simulink model "PC_CONTROL_STATION"  (R2023b)
settings: Solver=FixedStepAuto  StartTime=0.0  StopTime=inf  RelTol=1e-3  EnableMultiTasking=on
InitFcn:
  | if RUN_MODE~=5
  |     % clear rpi;
  |     rpi = raspberrypi(CAR_IP, 'pi', 'LabControl');
  |     stopModel(rpi,'CAR_CONTROL_SYSTEM')
  |     while isModelRunning(rpi,'CAR_CONTROL_SYSTEM')
  |          stopModel(rpi,'CAR_CONTROL_SYSTEM')
  |     end
  |     runModel(rpi,'CAR_CONTROL_SYSTEM')
  |      while isModelRunning(rpi,'CAR_CONTROL_SYSTEM')==false
  |          runModel(rpi,'CAR_CONTROL_SYSTEM')
  |      end
  |      % clear rpi;
  | end
StopFcn:
  | if RUN_MODE~=5
  |    clear rpi;
  |    rpi = raspberrypi(CAR_IP, 'pi', 'LabControl');
  |    stopModel(rpi,'CAR_CONTROL_SYSTEM')
  |    while isModelRunning(rpi,'CAR_CONTROL_SYSTEM')
  |    end
  |    clear rpi;
  | end
model workspace (MAT data in the model file):
  SL_ROS_VariableLengthArrays_MaxSizes : object (value not decoded)
values from neighbouring files (symbols this model uses):
  data = theClient.GetLastFrameOfData()    [FuncMotive.m]
undefined symbols (not defined in the file or in its folder): CONTROL, CONTROL_INI, data_SL_Info, MD25, MSG, SAMPLING_TIME, Standard_Devices, SYSID_INPUT, TCP_Protocol, UDP_Protocol
libraries: simulink x51, sldrtlib x46, dspsigattribs x7, ros2lib x3, ctrlSharedLib x2, aerolibanimutils x1
(part 2 of 8)

== system PC_CONTROL_STATION/HARDWARE/RT_MONITORING/TCP 106 ==
  Compare To Zero : simulink/Logic and Bit Operations/Compare To Zero  relop=>  OutDataTypeStr=boolean
  Data Store Read : DataStoreRead  DataStoreName=MSG  SampleTime=CONTROL_INI.PARAM.COMM_SAMPLING_TIME  DataStoreElements=MSG.TX_BUFFER(1,1)  IndexOptions=Index vector (dialog)  Indices=1  OutputSizes=1
  MSG_RX : Subsystem  Priority=10
      settings: RTWSystemCode=Nonreusable function  FunctionWithSeparateData=on
  "MSG_TX " : Subsystem  Priority=10
      settings: RTWSystemCode=Nonreusable function  FunctionWithSeparateData=on
  wires:
  Compare To Zero/1 -> "MSG_TX "/Enable
  Data Store Read/1 -> Compare To Zero/1

== system PC_CONTROL_STATION/HARDWARE/RT_MONITORING/TCP 107 ==
  Compare To Zero : simulink/Logic and Bit Operations/Compare To Zero  relop=>  OutDataTypeStr=boolean
  Data Store Read : DataStoreRead  DataStoreName=MSG  SampleTime=CONTROL_INI.PARAM.COMM_SAMPLING_TIME  DataStoreElements=MSG.TX_BUFFER(1,1)  IndexOptions=Index vector (dialog)  Indices=1  OutputSizes=1
  MSG_RX : Subsystem  Priority=10
      settings: RTWSystemCode=Nonreusable function  FunctionWithSeparateData=on
  "MSG_TX " : Subsystem  Priority=10
      settings: RTWSystemCode=Nonreusable function  FunctionWithSeparateData=on
  wires:
  Compare To Zero/1 -> "MSG_TX "/Enable
  Data Store Read/1 -> Compare To Zero/1

== system PC_CONTROL_STATION/HARDWARE/RT_MONITORING/TCP 108 ==
  Compare To Zero : simulink/Logic and Bit Operations/Compare To Zero  relop=>  OutDataTypeStr=boolean
  Data Store Read : DataStoreRead  DataStoreName=MSG  SampleTime=CONTROL_INI.PARAM.COMM_SAMPLING_TIME  DataStoreElements=MSG.TX_BUFFER(1,1)  IndexOptions=Index vector (dialog)  Indices=1  OutputSizes=1
  MSG_RX : Subsystem  Priority=10
      settings: RTWSystemCode=Nonreusable function  FunctionWithSeparateData=on
  "MSG_TX " : Subsystem  Priority=10
      settings: RTWSystemCode=Nonreusable function  FunctionWithSeparateData=on
  wires:
  Compare To Zero/1 -> "MSG_TX "/Enable
  Data Store Read/1 -> Compare To Zero/1

== system PC_CONTROL_STATION/HARDWARE/RT_MONITORING/TCP 109 ==
  Compare To Zero : simulink/Logic and Bit Operations/Compare To Zero  relop=>  OutDataTypeStr=boolean
  Data Store Read : DataStoreRead  DataStoreName=MSG  SampleTime=CONTROL_INI.PARAM.COMM_SAMPLING_TIME  DataStoreElements=MSG.TX_BUFFER(1,1)  IndexOptions=Index vector (dialog)  Indices=1  OutputSizes=1
  MSG_RX : Subsystem  Priority=10
      settings: RTWSystemCode=Nonreusable function  FunctionWithSeparateData=on
  "MSG_TX " : Subsystem  Priority=10
      settings: RTWSystemCode=Nonreusable function  FunctionWithSeparateData=on
  wires:
  Compare To Zero/1 -> "MSG_TX "/Enable
  Data Store Read/1 -> Compare To Zero/1

== system PC_CONTROL_STATION/HARDWARE/RT_MONITORING/TCP 110 ==
  Compare To Zero : simulink/Logic and Bit Operations/Compare To Zero  relop=>  OutDataTypeStr=boolean
  Data Store Read : DataStoreRead  DataStoreName=MSG  SampleTime=CONTROL_INI.PARAM.COMM_SAMPLING_TIME  DataStoreElements=MSG.TX_BUFFER(1,1)  IndexOptions=Index vector (dialog)  Indices=1  OutputSizes=1
  MSG_RX : Subsystem  Priority=10
      settings: RTWSystemCode=Nonreusable function  FunctionWithSeparateData=on
  "MSG_TX " : Subsystem  Priority=10
      settings: RTWSystemCode=Nonreusable function  FunctionWithSeparateData=on
  wires:
  Compare To Zero/1 -> "MSG_TX "/Enable
  Data Store Read/1 -> Compare To Zero/1

== system PC_CONTROL_STATION/HARDWARE/RT_MONITORING/TCP 111 ==
  Compare To Zero : simulink/Logic and Bit Operations/Compare To Zero  relop=>  OutDataTypeStr=boolean
  Data Store Read : DataStoreRead  DataStoreName=MSG  SampleTime=CONTROL_INI.PARAM.COMM_SAMPLING_TIME  DataStoreElements=MSG.TX_BUFFER(1,1)  IndexOptions=Index vector (dialog)  Indices=1  OutputSizes=1
  MSG_RX : Subsystem  Priority=10
      settings: RTWSystemCode=Nonreusable function  FunctionWithSeparateData=on
  "MSG_TX " : Subsystem  Priority=10
      settings: RTWSystemCode=Nonreusable function  FunctionWithSeparateData=on
  wires:
  Compare To Zero/1 -> "MSG_TX "/Enable
  Data Store Read/1 -> Compare To Zero/1

== system PC_CONTROL_STATION/HARDWARE/RT_MONITORING/TCP 112 ==
  Compare To Zero : simulink/Logic and Bit Operations/Compare To Zero  relop=>  OutDataTypeStr=boolean
  Data Store Read : DataStoreRead  DataStoreName=MSG  SampleTime=CONTROL_INI.PARAM.COMM_SAMPLING_TIME  DataStoreElements=MSG.TX_BUFFER(1,1)  IndexOptions=Index vector (dialog)  Indices=1  OutputSizes=1
  MSG_RX : Subsystem  Priority=10
      settings: RTWSystemCode=Nonreusable function  FunctionWithSeparateData=on
  "MSG_TX " : Subsystem  Priority=10
      settings: RTWSystemCode=Nonreusable function  FunctionWithSeparateData=on
  wires:
  Compare To Zero/1 -> "MSG_TX "/Enable
  Data Store Read/1 -> Compare To Zero/1

== system PC_CONTROL_STATION/HARDWARE/RT_MONITORING/TCP 113 ==
  Compare To Zero : simulink/Logic and Bit Operations/Compare To Zero  relop=>  OutDataTypeStr=boolean
  Data Store Read : DataStoreRead  DataStoreName=MSG  SampleTime=CONTROL_INI.PARAM.COMM_SAMPLING_TIME  DataStoreElements=MSG.TX_BUFFER(1,1)  IndexOptions=Index vector (dialog)  Indices=1  OutputSizes=1
  MSG_RX : Subsystem  Priority=10
      settings: RTWSystemCode=Nonreusable function  FunctionWithSeparateData=on
  "MSG_TX " : Subsystem  Priority=10
      settings: RTWSystemCode=Nonreusable function  FunctionWithSeparateData=on
  wires:
  Compare To Zero/1 -> "MSG_TX "/Enable
  Data Store Read/1 -> Compare To Zero/1

== system PC_CONTROL_STATION/HARDWARE/RT_MONITORING/TCP 114 ==
  Compare To Zero : simulink/Logic and Bit Operations/Compare To Zero  relop=>  OutDataTypeStr=boolean
  Data Store Read : DataStoreRead  DataStoreName=MSG  SampleTime=CONTROL_INI.PARAM.COMM_SAMPLING_TIME  DataStoreElements=MSG.TX_BUFFER(1,1)  IndexOptions=Index vector (dialog)  Indices=1  OutputSizes=1
  MSG_RX : Subsystem  Priority=10
      settings: RTWSystemCode=Nonreusable function  FunctionWithSeparateData=on
  "MSG_TX " : Subsystem  Priority=10
      settings: RTWSystemCode=Nonreusable function  FunctionWithSeparateData=on
  wires:
  Compare To Zero/1 -> "MSG_TX "/Enable
  Data Store Read/1 -> Compare To Zero/1

== system PC_CONTROL_STATION/HARDWARE/RT_MONITORING/TCP 115 ==
  Compare To Zero : simulink/Logic and Bit Operations/Compare To Zero  relop=>  OutDataTypeStr=boolean
  Data Store Read : DataStoreRead  DataStoreName=MSG  SampleTime=CONTROL_INI.PARAM.COMM_SAMPLING_TIME  DataStoreElements=MSG.TX_BUFFER(1,1)  IndexOptions=Index vector (dialog)  Indices=1  OutputSizes=1
  MSG_RX : Subsystem  Priority=10
      settings: RTWSystemCode=Nonreusable function  FunctionWithSeparateData=on
  "MSG_TX " : Subsystem  Priority=10
      settings: RTWSystemCode=Nonreusable function  FunctionWithSeparateData=on
  wires:
  Compare To Zero/1 -> "MSG_TX "/Enable
  Data Store Read/1 -> Compare To Zero/1

== system PC_CONTROL_STATION/HARDWARE/RT_MONITORING/TCP 116 ==
  Compare To Zero : simulink/Logic and Bit Operations/Compare To Zero  relop=>  OutDataTypeStr=boolean
  Data Store Read : DataStoreRead  DataStoreName=MSG  SampleTime=CONTROL_INI.PARAM.COMM_SAMPLING_TIME  DataStoreElements=MSG.TX_BUFFER(1,1)  IndexOptions=Index vector (dialog)  Indices=1  OutputSizes=1
  MSG_RX : Subsystem  Priority=10
      settings: RTWSystemCode=Nonreusable function  FunctionWithSeparateData=on
  "MSG_TX " : Subsystem  Priority=10
      settings: RTWSystemCode=Nonreusable function  FunctionWithSeparateData=on
  wires:
  Compare To Zero/1 -> "MSG_TX "/Enable
  Data Store Read/1 -> Compare To Zero/1

== system PC_CONTROL_STATION/HARDWARE/RT_MONITORING/TCP 117 ==
  Compare To Zero : simulink/Logic and Bit Operations/Compare To Zero  relop=>  OutDataTypeStr=boolean
  Data Store Read : DataStoreRead  DataStoreName=MSG  SampleTime=CONTROL_INI.PARAM.COMM_SAMPLING_TIME  DataStoreElements=MSG.TX_BUFFER(1,1)  IndexOptions=Index vector (dialog)  Indices=1  OutputSizes=1
  MSG_RX : Subsystem  Priority=10
      settings: RTWSystemCode=Nonreusable function  FunctionWithSeparateData=on
  "MSG_TX " : Subsystem  Priority=10
      settings: RTWSystemCode=Nonreusable function  FunctionWithSeparateData=on
  wires:
  Compare To Zero/1 -> "MSG_TX "/Enable
  Data Store Read/1 -> Compare To Zero/1

== system PC_CONTROL_STATION/HARDWARE/RT_MONITORING/TCP 118 ==
  Compare To Zero : simulink/Logic and Bit Operations/Compare To Zero  relop=>  OutDataTypeStr=boolean
  Data Store Read : DataStoreRead  DataStoreName=MSG  SampleTime=CONTROL_INI.PARAM.COMM_SAMPLING_TIME  DataStoreElements=MSG.TX_BUFFER(1,1)  IndexOptions=Index vector (dialog)  Indices=1  OutputSizes=1
  MSG_RX : Subsystem  Priority=10
      settings: RTWSystemCode=Nonreusable function  FunctionWithSeparateData=on
  "MSG_TX " : Subsystem  Priority=10
      settings: RTWSystemCode=Nonreusable function  FunctionWithSeparateData=on
  wires:
  Compare To Zero/1 -> "MSG_TX "/Enable
  Data Store Read/1 -> Compare To Zero/1

== system PC_CONTROL_STATION/HARDWARE/RT_MONITORING/TCP 119 ==
  Compare To Zero : simulink/Logic and Bit Operations/Compare To Zero  relop=>  OutDataTypeStr=boolean
  Data Store Read : DataStoreRead  DataStoreName=MSG  SampleTime=CONTROL_INI.PARAM.COMM_SAMPLING_TIME  DataStoreElements=MSG.TX_BUFFER(1,1)  IndexOptions=Index vector (dialog)  Indices=1  OutputSizes=1
  MSG_RX : Subsystem  Priority=10
      settings: RTWSystemCode=Nonreusable function  FunctionWithSeparateData=on
  "MSG_TX " : Subsystem  Priority=10
      settings: RTWSystemCode=Nonreusable function  FunctionWithSeparateData=on
  wires:
  Compare To Zero/1 -> "MSG_TX "/Enable
  Data Store Read/1 -> Compare To Zero/1

== system PC_CONTROL_STATION/HARDWARE/RT_MONITORING/TCP 120 ==
  Compare To Zero : simulink/Logic and Bit Operations/Compare To Zero  relop=>  OutDataTypeStr=boolean
  Data Store Read : DataStoreRead  DataStoreName=MSG  SampleTime=CONTROL_INI.PARAM.COMM_SAMPLING_TIME  DataStoreElements=MSG.TX_BUFFER(1,1)  IndexOptions=Index vector (dialog)  Indices=1  OutputSizes=1
  MSG_RX : Subsystem  Priority=10
      settings: RTWSystemCode=Nonreusable function  FunctionWithSeparateData=on
  "MSG_TX " : Subsystem  Priority=10
      settings: RTWSystemCode=Nonreusable function  FunctionWithSeparateData=on
  wires:
  Compare To Zero/1 -> "MSG_TX "/Enable
  Data Store Read/1 -> Compare To Zero/1

== system PC_CONTROL_STATION/HARDWARE/RT_MONITORING/TCP 121 ==
  Compare To Zero : simulink/Logic and Bit Operations/Compare To Zero  relop=>  OutDataTypeStr=boolean
  Data Store Read : DataStoreRead  DataStoreName=MSG  SampleTime=CONTROL_INI.PARAM.COMM_SAMPLING_TIME  DataStoreElements=MSG.TX_BUFFER(1,1)  IndexOptions=Index vector (dialog)  Indices=1  OutputSizes=1
  MSG_RX : Subsystem  Priority=10
      settings: RTWSystemCode=Nonreusable function  FunctionWithSeparateData=on
  "MSG_TX " : Subsystem  Priority=10
      settings: RTWSystemCode=Nonreusable function  FunctionWithSeparateData=on
  wires:
  Compare To Zero/1 -> "MSG_TX "/Enable
  Data Store Read/1 -> Compare To Zero/1

== system PC_CONTROL_STATION/HARDWARE/RT_MONITORING/TCP RSP ==
  Compare To Zero : simulink/Logic and Bit Operations/Compare To Zero  relop=>  OutDataTypeStr=boolean
  Data Store Read : DataStoreRead  DataStoreName=MSG  SampleTime=CONTROL_INI.PARAM.COMM_SAMPLING_TIME  DataStoreElements=MSG.TX_BUFFER(1,1)  IndexOptions=Index vector (dialog)  Indices=1  OutputSizes=1
  MSG_RX : Subsystem  Priority=10
      settings: RTWSystemCode=Nonreusable function  FunctionWithSeparateData=on
  "MSG_TX " : Subsystem  Priority=10
      settings: RTWSystemCode=Nonreusable function  FunctionWithSeparateData=on
  wires:
  Compare To Zero/1 -> "MSG_TX "/Enable
  Data Store Read/1 -> Compare To Zero/1

== system PC_CONTROL_STATION/HARDWARE/RT_MONITORING/UDP ==
  Compare To Zero : simulink/Logic and Bit Operations/Compare To Zero  relop=>  OutDataTypeStr=boolean
  Data Store Read : DataStoreRead  DataStoreName=MSG  SampleTime=CONTROL_INI.PARAM.COMM_SAMPLING_TIME  DataStoreElements=MSG.TX_BUFFER(1,1)  IndexOptions=Index vector (dialog)  Indices=1  OutputSizes=1
  MSG_RX : Subsystem  Priority=10
      settings: RTWSystemCode=Nonreusable function  FunctionWithSeparateData=on
  "MSG_TX " : Subsystem  Priority=10
      settings: RTWSystemCode=Nonreusable function  FunctionWithSeparateData=on
  wires:
  Compare To Zero/1 -> "MSG_TX "/Enable
  Data Store Read/1 -> Compare To Zero/1

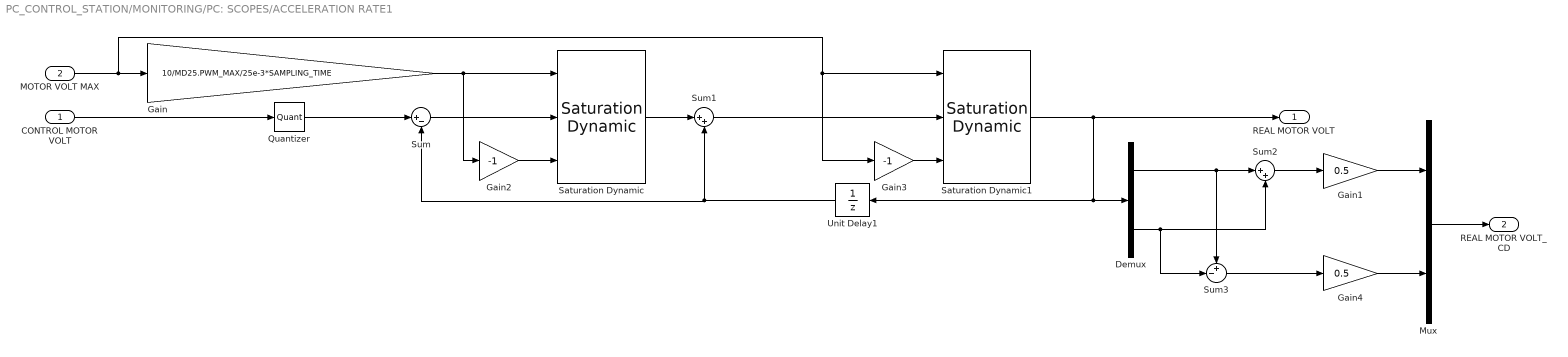
== system PC_CONTROL_STATION/MONITORING/PC: SCOPES/ACCELERATION RATE1 ==
  CONTROL MOTOR VOLT : Inport
  MOTOR VOLT MAX : Inport  Port=2
  Demux : Demux  Outputs=2
  Gain : Gain  Gain=10/MD25.PWM_MAX/25e-3*SAMPLING_TIME
  Gain1 : Gain  Gain=0.5
  Gain2 : Gain  Gain=-1
  Gain3 : Gain  Gain=-1
  Gain4 : Gain  Gain=0.5
  Mux : Mux  Inputs=2
  Quantizer : Quantizer  QuantizationInterval=CONTROL_INI.PARAM.MOTOR_VOLT_MAX(1)/127
  Saturation Dynamic : simulink/Discontinuities/Saturation Dynamic  OutMin=[]  OutMax=[]  OutDataTypeStr=Inherit: Same as second input  OutDataType=fixdt(1, 16)  OutScaling=2^-10  DoSatur=off
  Saturation Dynamic1 : simulink/Discontinuities/Saturation Dynamic  OutMin=[]  OutMax=[]  OutDataTypeStr=Inherit: Same as second input  OutDataType=fixdt(1, 16)  OutScaling=2^-10  DoSatur=off
  Sum : Sum  Inputs=|+-
  Sum1 : Sum  Inputs=|++
  Sum2 : Sum  Inputs=|++
  Sum3 : Sum  Inputs=+-|
  Unit Delay1 : UnitDelay  SampleTime=-1  HasFrameUpgradeWarning=on
  REAL MOTOR VOLT : Outport
  REAL MOTOR VOLT_CD : Outport  Port=2
  wires:
  CONTROL MOTOR VOLT/1 -> Quantizer/1
  Gain3/1 -> Saturation Dynamic1/3
  Gain2/1 -> Saturation Dynamic/3
  Sum/1 -> Saturation Dynamic/2
  MOTOR VOLT MAX/1 -> Gain/1, Gain3/1, Saturation Dynamic1/1
  Sum1/1 -> Saturation Dynamic1/2
  Gain/1 -> Gain2/1, Saturation Dynamic/1
  Saturation Dynamic/1 -> Sum1/1
  Saturation Dynamic1/1 -> Unit Delay1/1, Demux/1, REAL MOTOR VOLT/1
  Demux/1 -> Sum3/1, Sum2/1
  Demux/2 -> Sum3/2, Sum2/2
  Sum2/1 -> Gain1/1
  Sum3/1 -> Gain4/1
  Gain1/1 -> Mux/1
  Gain4/1 -> Mux/2
  Mux/1 -> REAL MOTOR VOLT_CD/1
  Unit Delay1/1 -> Sum/2, Sum1/2
  Quantizer/1 -> Sum/1

== system PC_CONTROL_STATION/MONITORING/SYSTEM IDENTIFICATION/STATE VARIABLE FILTER 1 ==
  IN : Inport
  Add : Sum  Inputs=3
  Constant : Constant  Value=SVF_B1d  SampleTime=SAMPLING_TIME
  Constant1 : Constant  Value=SVF_B2d  SampleTime=SAMPLING_TIME
  Constant2 : Constant  Value=SVF_Ad  SampleTime=SAMPLING_TIME
  Divide : Product  Multiplication=Matrix(*)
  Divide1 : Product  Multiplication=Matrix(*)
  Divide2 : Product  Multiplication=Matrix(*)
  Unit Delay : UnitDelay  InitialCondition=zeros(4,1)  SampleTime=-1  HasFrameUpgradeWarning=on
  Unit Delay1 : UnitDelay  SampleTime=-1  HasFrameUpgradeWarning=on
  STATE : Outport  VectorParamsAs1DForOutWhenUnconnected=off
  wires:
  Constant/1 -> Divide1/1
  Unit Delay1/1 -> Divide1/2
  Divide1/1 -> Add/1
  Add/1 -> STATE/1, Unit Delay/1
  Divide/1 -> Add/2
  Constant1/1 -> Divide/1
  Divide2/1 -> Add/3
  Constant2/1 -> Divide2/1
  Unit Delay/1 -> Divide2/2
  IN/1 -> Divide/2, Unit Delay1/1

== system PC_CONTROL_STATION/MONITORING/SYSTEM IDENTIFICATION/STATE VARIABLE FILTER 2 ==
  IN : Inport
  Add : Sum  Inputs=3
  Constant : Constant  Value=SVF_B1d  SampleTime=SAMPLING_TIME
  Constant1 : Constant  Value=SVF_B2d  SampleTime=SAMPLING_TIME
  Constant2 : Constant  Value=SVF_Ad  SampleTime=SAMPLING_TIME
  Divide : Product  Multiplication=Matrix(*)
  Divide1 : Product  Multiplication=Matrix(*)
  Divide2 : Product  Multiplication=Matrix(*)
  Unit Delay : UnitDelay  InitialCondition=zeros(4,1)  SampleTime=-1  HasFrameUpgradeWarning=on
  Unit Delay1 : UnitDelay  SampleTime=-1  HasFrameUpgradeWarning=on
  STATE : Outport  VectorParamsAs1DForOutWhenUnconnected=off
  wires:
  IN/1 -> Unit Delay1/1, Divide/2
  Unit Delay/1 -> Divide2/2
  Constant2/1 -> Divide2/1
  Divide2/1 -> Add/3
  Constant1/1 -> Divide/1
  Divide/1 -> Add/2
  Add/1 -> Unit Delay/1, STATE/1
  Divide1/1 -> Add/1
  Unit Delay1/1 -> Divide1/2
  Constant/1 -> Divide1/1

== system PC_CONTROL_STATION/MONITORING/SYSTEM IDENTIFICATION/STATE VARIABLE FILTER 3 ==
  IN : Inport
  Add : Sum  Inputs=3
  Constant : Constant  Value=SVF_B1d  SampleTime=SAMPLING_TIME
  Constant1 : Constant  Value=SVF_B2d  SampleTime=SAMPLING_TIME
  Constant2 : Constant  Value=SVF_Ad  SampleTime=SAMPLING_TIME
  Divide : Product  Multiplication=Matrix(*)
  Divide1 : Product  Multiplication=Matrix(*)
  Divide2 : Product  Multiplication=Matrix(*)
  Unit Delay : UnitDelay  InitialCondition=zeros(4,1)  SampleTime=-1  HasFrameUpgradeWarning=on
  Unit Delay1 : UnitDelay  SampleTime=-1  HasFrameUpgradeWarning=on
  STATE : Outport  VectorParamsAs1DForOutWhenUnconnected=off
  wires:
  Constant/1 -> Divide1/1
  Unit Delay1/1 -> Divide1/2
  Divide1/1 -> Add/1
  Add/1 -> STATE/1, Unit Delay/1
  Divide/1 -> Add/2
  Constant1/1 -> Divide/1
  Divide2/1 -> Add/3
  Constant2/1 -> Divide2/1
  Unit Delay/1 -> Divide2/2
  IN/1 -> Divide/2, Unit Delay1/1

== system PC_CONTROL_STATION/MONITORING/SYSTEM IDENTIFICATION/STATE VARIABLE FILTER 4 ==
  IN : Inport
  Add : Sum  Inputs=3
  Constant : Constant  Value=SVF_B1d  SampleTime=SAMPLING_TIME
  Constant1 : Constant  Value=SVF_B2d  SampleTime=SAMPLING_TIME
  Constant2 : Constant  Value=SVF_Ad  SampleTime=SAMPLING_TIME
  Divide : Product  Multiplication=Matrix(*)
  Divide1 : Product  Multiplication=Matrix(*)
  Divide2 : Product  Multiplication=Matrix(*)
  Unit Delay : UnitDelay  InitialCondition=zeros(4,1)  SampleTime=-1  HasFrameUpgradeWarning=on
  Unit Delay1 : UnitDelay  SampleTime=-1  HasFrameUpgradeWarning=on
  STATE : Outport  VectorParamsAs1DForOutWhenUnconnected=off
  wires:
  IN/1 -> Unit Delay1/1, Divide/2
  Unit Delay/1 -> Divide2/2
  Constant2/1 -> Divide2/1
  Divide2/1 -> Add/3
  Constant1/1 -> Divide/1
  Divide/1 -> Add/2
  Add/1 -> Unit Delay/1, STATE/1
  Divide1/1 -> Add/1
  Unit Delay1/1 -> Divide1/2
  Constant/1 -> Divide1/1

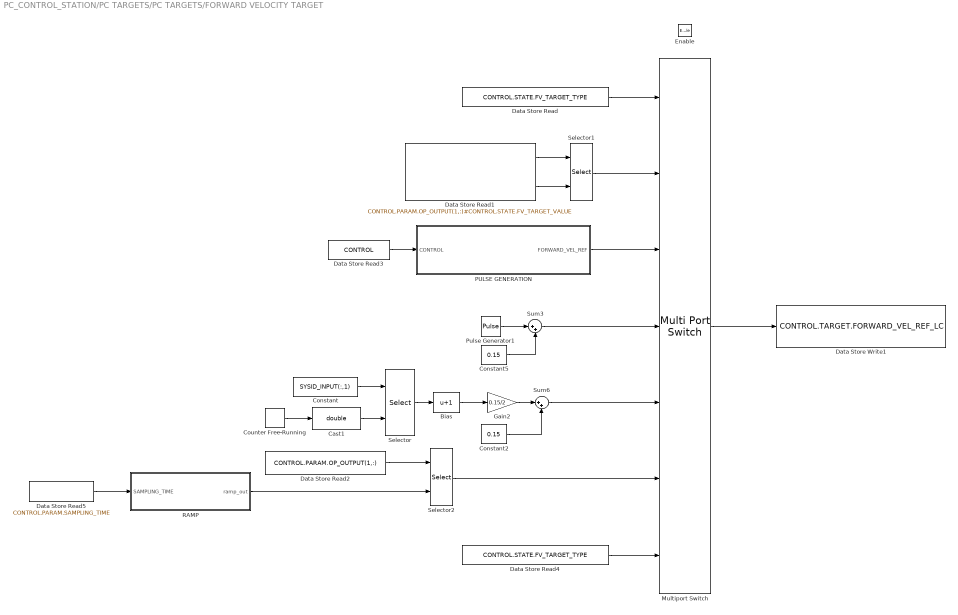
== system PC_CONTROL_STATION/PC TARGETS/PC TARGETS/FORWARD VELOCITY TARGET ==
  Enable : EnablePort
  " PULSE GENERATION" : MATLAB Function  Priority=60  TreatAsAtomicUnit=on
  Bias : Bias  Bias=1  SaturateOnIntegerOverflow=off
  Cast1 : DataTypeConversion  OutDataTypeStr=double  SaturateOnIntegerOverflow=off  RndMeth=Floor
  Constant : Constant  Value=SYSID_INPUT(:,1)  SampleTime=SAMPLING_TIME
  Constant2 : Constant  Value=0.15  OutDataTypeStr=double  SampleTime=SAMPLING_TIME
  Constant5 : Constant  Value=0.15  OutDataTypeStr=double  SampleTime=SAMPLING_TIME
  Counter Free-Running : simulink/Sources/Counter Free-Running  NumBits=9  tsamp=SAMPLING_TIME
  Data Store Read : DataStoreRead  DataStoreName=CONTROL  SampleTime=SAMPLING_TIME  DataStoreElements=CONTROL.STATE.FV_TARGET_TYPE  IndexOptions=Index vector (dialog)  Indices=1  OutputSizes=1
  Data Store Read1 : DataStoreRead  DataStoreName=CONTROL  SampleTime=SAMPLING_TIME  DataStoreElements=CONTROL.PARAM.OP_OUTPUT(1,:)#CONTROL.STATE.FV_TARGET_VALUE  IndexOptions=Index vector (dialog)  Indices=1  OutputSizes=1
  Data Store Read2 : DataStoreRead  DataStoreName=CONTROL  SampleTime=SAMPLING_TIME  DataStoreElements=CONTROL.PARAM.OP_OUTPUT(1,:)  IndexOptions=Index vector (dialog)  Indices=1  OutputSizes=1
  Data Store Read3 : DataStoreRead  DataStoreName=CONTROL  SampleTime=SAMPLING_TIME  IndexOptions=Index vector (dialog)  Indices=1  OutputSizes=1
  Data Store Read4 : DataStoreRead  DataStoreName=CONTROL  SampleTime=SAMPLING_TIME  DataStoreElements=CONTROL.STATE.FV_TARGET_TYPE  IndexOptions=Index vector (dialog)  Indices=1  OutputSizes=1
  Data Store Read5 : DataStoreRead  DataStoreName=CONTROL  SampleTime=SAMPLING_TIME  DataStoreElements=CONTROL.PARAM.SAMPLING_TIME  IndexOptions=Index vector (dialog)  Indices=1  OutputSizes=1
  Data Store Write1 : DataStoreWrite  DataStoreName=CONTROL  SampleTime=SAMPLING_TIME  DataStoreElements=CONTROL.TARGET.FORWARD_VEL_REF_LC  IndexOptions=Index vector (dialog)  Indices=1  OutputSizes=1
  Gain2 : Gain  Gain=0.15/2
  Multiport Switch : MultiPortSwitch  DataPortOrder=Zero-based contiguous  Inputs=6  zeroidx=on  SaturateOnIntegerOverflow=off  InputSameDT=off
  Pulse Generator1 : DiscretePulseGenerator  Amplitude=0.15  Period=500  PulseWidth=250  SampleTime=SAMPLING_TIME
  RAMP : MATLAB Function  TreatAsAtomicUnit=on
  Selector : Selector  IndexMode=Zero-based  InputPortWidth=512  IndexOptions=Index vector (port)  Indices=[1 3]  OutputSizes=1
  Selector1 : Selector  InputPortWidth=4  IndexOptions=Index vector (port)  Indices=[1 3]  OutputSizes=1
  Selector2 : Selector  InputPortWidth=4  IndexOptions=Index vector (port)  Indices=[1 3]  OutputSizes=1
  Sum3 : Sum  Inputs=|++
  Sum6 : Sum  Inputs=|++
  wires:
  Constant5/1 -> Sum3/2
  Pulse Generator1/1 -> Sum3/1
  Counter Free-Running/1 -> Cast1/1
  Sum6/1 -> Multiport Switch/5
  Sum3/1 -> Multiport Switch/4
  Gain2/1 -> Sum6/1
  Selector1/1 -> Multiport Switch/2
  Constant/1 -> Selector/1
  Data Store Read/1 -> Multiport Switch/1
  Cast1/1 -> Selector/2
  Constant2/1 -> Sum6/2
  Multiport Switch/1 -> Data Store Write1/1
  Data Store Read3/1 -> " PULSE GENERATION"/1(CONTROL)
  " PULSE GENERATION"/1(FORWARD_VEL_REF) -> Multiport Switch/3
  Data Store Read1/1 -> Selector1/1
  Data Store Read1/2 -> Selector1/2
  Selector2/1 -> Multiport Switch/6
  Data Store Read2/1 -> Selector2/1
  Data Store Read4/1 -> Multiport Switch/7
  RAMP/1(ramp_out) -> Selector2/2
  Data Store Read5/1 -> RAMP/1(SAMPLING_TIME)
  Selector/1 -> Bias/1
  Bias/1 -> Gain2/1

== system PC_CONTROL_STATION/PC TARGETS/PC TARGETS/NAVIGATION TARGETS ==
  Enable : EnablePort
  Data Store Read7 : DataStoreRead  DataStoreName=CONTROL  SampleTime=SAMPLING_TIME  IndexOptions=Index vector (dialog)  Indices=1  OutputSizes=1
  Data Store Write : DataStoreWrite  DataStoreName=CONTROL  SampleTime=SAMPLING_TIME  IndexOptions=Index vector (dialog)  Indices=1  OutputSizes=1
  TRAJECTORY PLANNER (POLYNOMIAL IN Vx & Vy) : MATLAB Function  Priority=10  TreatAsAtomicUnit=on
  wires:
  Data Store Read7/1 -> TRAJECTORY PLANNER (POLYNOMIAL IN Vx & Vy)/1(CONTROL_IN)
  TRAJECTORY PLANNER (POLYNOMIAL IN Vx & Vy)/1(CONTROL) -> Data Store Write/1

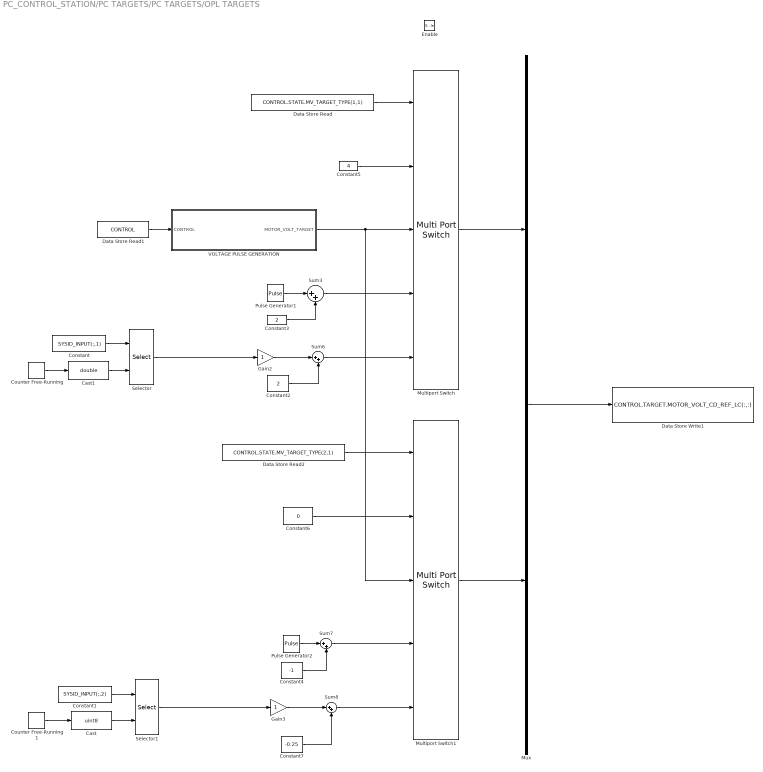
== system PC_CONTROL_STATION/PC TARGETS/PC TARGETS/OPL TARGETS ==
  Enable : EnablePort
  Cast : DataTypeConversion  OutDataTypeStr=uint8  SaturateOnIntegerOverflow=off  RndMeth=Floor
  Cast1 : DataTypeConversion  OutDataTypeStr=double  SaturateOnIntegerOverflow=off  RndMeth=Floor
  Constant : Constant  Value=SYSID_INPUT(:,1)  SampleTime=SAMPLING_TIME
  Constant1 : Constant  Value=SYSID_INPUT(:,2)  SampleTime=SAMPLING_TIME
  Constant2 : Constant  Value=2  OutDataTypeStr=single  SampleTime=SAMPLING_TIME
  Constant3 : Constant  Value=2  OutDataTypeStr=double  SampleTime=SAMPLING_TIME
  Constant4 : Constant  Value=-1  OutDataTypeStr=single  SampleTime=SAMPLING_TIME
  Constant5 : Constant  Value=4  OutDataTypeStr=double  SampleTime=SAMPLING_TIME
  Constant6 : Constant  Value=0  OutDataTypeStr=double  SampleTime=SAMPLING_TIME
  Constant7 : Constant  Value=-0.25  OutDataTypeStr=single  SampleTime=SAMPLING_TIME
  Counter Free-Running : simulink/Sources/Counter Free-Running  NumBits=9  tsamp=SAMPLING_TIME
  Counter Free-Running1 : simulink/Sources/Counter Free-Running  NumBits=9  tsamp=SAMPLING_TIME
  Data Store Read : DataStoreRead  DataStoreName=CONTROL  SampleTime=SAMPLING_TIME  DataStoreElements=CONTROL.STATE.MV_TARGET_TYPE(1,1)  IndexOptions=Index vector (dialog)  Indices=1  OutputSizes=1
  Data Store Read1 : DataStoreRead  DataStoreName=CONTROL  SampleTime=SAMPLING_TIME  IndexOptions=Index vector (dialog)  Indices=1  OutputSizes=1
  Data Store Read2 : DataStoreRead  DataStoreName=CONTROL  SampleTime=SAMPLING_TIME  DataStoreElements=CONTROL.STATE.MV_TARGET_TYPE(2,1)  IndexOptions=Index vector (dialog)  Indices=1  OutputSizes=1
  Data Store Write1 : DataStoreWrite  DataStoreName=CONTROL  SampleTime=SAMPLING_TIME  DataStoreElements=CONTROL.TARGET.MOTOR_VOLT_CD_REF_LC(:,:)  IndexOptions=Index vector (dialog)  Indices=1  OutputSizes=1
  Gain2 : Gain
  Gain3 : Gain
  Multiport Switch : MultiPortSwitch  DataPortOrder=Zero-based contiguous  Inputs=4  zeroidx=on  SaturateOnIntegerOverflow=off  InputSameDT=off
  Multiport Switch1 : MultiPortSwitch  DataPortOrder=Zero-based contiguous  Inputs=4  zeroidx=on  SaturateOnIntegerOverflow=off  InputSameDT=off
  Mux : Mux  Inputs=2
  Pulse Generator1 : DiscretePulseGenerator  Amplitude=2  Period=200  PulseWidth=100  SampleTime=SAMPLING_TIME
  Pulse Generator2 : DiscretePulseGenerator  Amplitude=2  Period=200  PulseWidth=100  SampleTime=SAMPLING_TIME
  Selector : Selector  IndexMode=Zero-based  InputPortWidth=512  IndexOptions=Index vector (port)  Indices=[1 3]  OutputSizes=1
  Selector1 : Selector  IndexMode=Zero-based  InputPortWidth=512  IndexOptions=Index vector (port)  Indices=[1 3]  OutputSizes=1
  Sum{3,6..8} (4 alike) : Sum  Inputs=|++
  VOLTAGE PULSE GENERATION : MATLAB Function  Priority=60  TreatAsAtomicUnit=on
  wires:
  VOLTAGE PULSE GENERATION/1(MOTOR_VOLT_TARGET) -> Multiport Switch/3, Multiport Switch1/3
  Constant6/1 -> Multiport Switch1/2
  Constant7/1 -> Sum8/2
  Sum6/1 -> Multiport Switch/5
  Mux/1 -> Data Store Write1/1
  Sum3/1 -> Multiport Switch/4
  Gain2/1 -> Sum6/1
  Counter Free-Running/1 -> Cast1/1
  Cast1/1 -> Selector/2
  Sum8/1 -> Multiport Switch1/5
  Sum7/1 -> Multiport Switch1/4
  Selector1/1 -> Gain3/1
  Multiport Switch1/1 -> Mux/2
  Constant1/1 -> Selector1/1
  Constant/1 -> Selector/1
  Constant4/1 -> Sum7/2
  Gain3/1 -> Sum8/1
  Multiport Switch/1 -> Mux/1
  Data Store Read2/1 -> Multiport Switch1/1
  Cast/1 -> Selector1/2
  Constant2/1 -> Sum6/2
  Selector/1 -> Gain2/1
  Pulse Generator2/1 -> Sum7/1
  Counter Free-Running1/1 -> Cast/1
  Data Store Read/1 -> Multiport Switch/1
  Data Store Read1/1 -> VOLTAGE PULSE GENERATION/1(CONTROL)
  Constant5/1 -> Multiport Switch/2
  Pulse Generator1/1 -> Sum3/1
  Constant3/1 -> Sum3/2

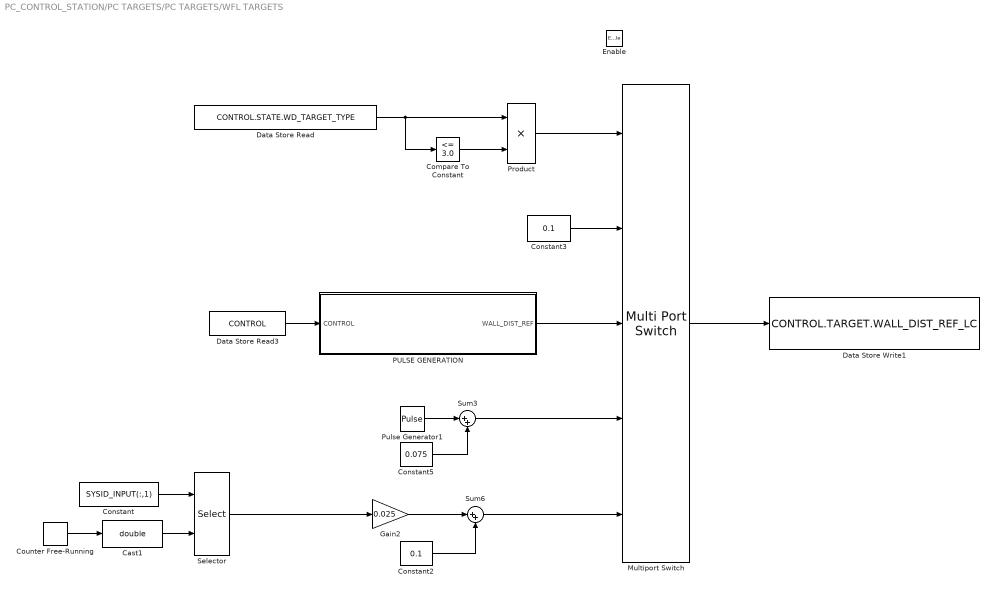
== system PC_CONTROL_STATION/PC TARGETS/PC TARGETS/WFL TARGETS ==
  Enable : EnablePort
  " PULSE GENERATION" : MATLAB Function  Priority=60  TreatAsAtomicUnit=on
  Cast1 : DataTypeConversion  OutDataTypeStr=double  SaturateOnIntegerOverflow=off  RndMeth=Floor
  Compare To Constant : simulink/Logic and Bit Operations/Compare To Constant  relop=<=  const=3.0  OutDataTypeStr=uint8
  Constant : Constant  Value=SYSID_INPUT(:,1)  SampleTime=SAMPLING_TIME
  Constant2 : Constant  Value=0.1  OutDataTypeStr=single  SampleTime=SAMPLING_TIME
  Constant3 : Constant  Value=0.1  OutDataTypeStr=double  SampleTime=SAMPLING_TIME
  Constant5 : Constant  Value=0.075  OutDataTypeStr=single  SampleTime=SAMPLING_TIME
  Counter Free-Running : simulink/Sources/Counter Free-Running  NumBits=9  tsamp=SAMPLING_TIME
  Data Store Read : DataStoreRead  DataStoreName=CONTROL  SampleTime=SAMPLING_TIME  DataStoreElements=CONTROL.STATE.WD_TARGET_TYPE  IndexOptions=Index vector (dialog)  Indices=1  OutputSizes=1
  Data Store Read3 : DataStoreRead  DataStoreName=CONTROL  SampleTime=SAMPLING_TIME  IndexOptions=Index vector (dialog)  Indices=1  OutputSizes=1
  Data Store Write1 : DataStoreWrite  DataStoreName=CONTROL  SampleTime=SAMPLING_TIME  DataStoreElements=CONTROL.TARGET.WALL_DIST_REF_LC  IndexOptions=Index vector (dialog)  Indices=1  OutputSizes=1
  Gain2 : Gain  Gain=0.025
  Multiport Switch : MultiPortSwitch  DataPortOrder=Zero-based contiguous  Inputs=4  zeroidx=on  SaturateOnIntegerOverflow=off  InputSameDT=off
  Product : Product
  Pulse Generator1 : DiscretePulseGenerator  Amplitude=0.025  Period=1000  PulseWidth=500  SampleTime=SAMPLING_TIME
  Selector : Selector  IndexMode=Zero-based  InputPortWidth=512  IndexOptions=Index vector (port)  Indices=[1 3]  OutputSizes=1
  Sum3 : Sum  Inputs=|++
  Sum6 : Sum  Inputs=|++
  wires:
  Pulse Generator1/1 -> Sum3/1
  Data Store Read3/1 -> " PULSE GENERATION"/1(CONTROL)
  Sum6/1 -> Multiport Switch/5
  Sum3/1 -> Multiport Switch/4
  Constant/1 -> Selector/1
  " PULSE GENERATION"/1(WALL_DIST_REF) -> Multiport Switch/3
  Constant2/1 -> Sum6/2
  Gain2/1 -> Sum6/1
  Constant5/1 -> Sum3/2
  Multiport Switch/1 -> Data Store Write1/1
  Cast1/1 -> Selector/2
  Constant3/1 -> Multiport Switch/2
  Selector/1 -> Gain2/1
  Counter Free-Running/1 -> Cast1/1
  Product/1 -> Multiport Switch/1
  Data Store Read/1 -> Compare To Constant/1, Product/1
  Compare To Constant/1 -> Product/2

== system PC_CONTROL_STATION/PC TARGETS/PC TARGETS/YAW ANGLE TARGET ==
  Enable : EnablePort
  " PULSE GENERATION" : MATLAB Function  Priority=60  TreatAsAtomicUnit=on
  Cast1 : DataTypeConversion  OutDataTypeStr=double  SaturateOnIntegerOverflow=off  RndMeth=Floor
  Constant : Constant  Value=SYSID_INPUT(:,1)  SampleTime=SAMPLING_TIME
  Constant3 : Constant  Value=0  OutDataTypeStr=double  SampleTime=SAMPLING_TIME
  Constant5 : Constant  Value=-60*pi/180  OutDataTypeStr=single  SampleTime=SAMPLING_TIME
  Constant8 : Constant  Value=-60*pi/180  OutDataTypeStr=single  SampleTime=SAMPLING_TIME
  Counter Free-Running : simulink/Sources/Counter Free-Running  NumBits=9  tsamp=SAMPLING_TIME
  Data Store Read : DataStoreRead  DataStoreName=CONTROL  SampleTime=SAMPLING_TIME  DataStoreElements=CONTROL.STATE.YA_TARGET_TYPE  IndexOptions=Index vector (dialog)  Indices=1  OutputSizes=1
  Data Store Read1 : DataStoreRead  DataStoreName=CONTROL  SampleTime=SAMPLING_TIME  IndexOptions=Index vector (dialog)  Indices=1  OutputSizes=1
  Data Store Write1 : DataStoreWrite  DataStoreName=CONTROL  SampleTime=SAMPLING_TIME  DataStoreElements=CONTROL.TARGET.YAW_ANG_REF_LC  IndexOptions=Index vector (dialog)  Indices=1  OutputSizes=1
  Gain2 : Gain  Gain=120*pi/180
  Multiport Switch : MultiPortSwitch  DataPortOrder=Zero-based contiguous  Inputs=4  zeroidx=on  SaturateOnIntegerOverflow=off  InputSameDT=off
  Pulse Generator1 : DiscretePulseGenerator  Amplitude=120*pi/180  Period=500  PulseWidth=250  PhaseDelay=125  SampleTime=SAMPLING_TIME
  Selector : Selector  IndexMode=Zero-based  InputPortWidth=512  IndexOptions=Index vector (port)  Indices=[1 3]  OutputSizes=1
  Sum3 : Sum  Inputs=|++
  Sum6 : Sum  Inputs=|++
  wires:
  Constant5/1 -> Sum3/2
  Selector/1 -> Gain2/1
  Pulse Generator1/1 -> Sum3/1
  Counter Free-Running/1 -> Cast1/1
  Sum6/1 -> Multiport Switch/5
  " PULSE GENERATION"/1(YAW_ANG_REF) -> Multiport Switch/3
  Sum3/1 -> Multiport Switch/4
  Gain2/1 -> Sum6/1
  Constant3/1 -> Multiport Switch/2
  Constant/1 -> Selector/1
  Data Store Read/1 -> Multiport Switch/1
  Data Store Read1/1 -> " PULSE GENERATION"/1(CONTROL)
  Cast1/1 -> Selector/2
  Constant8/1 -> Sum6/2
  Multiport Switch/1 -> Data Store Write1/1

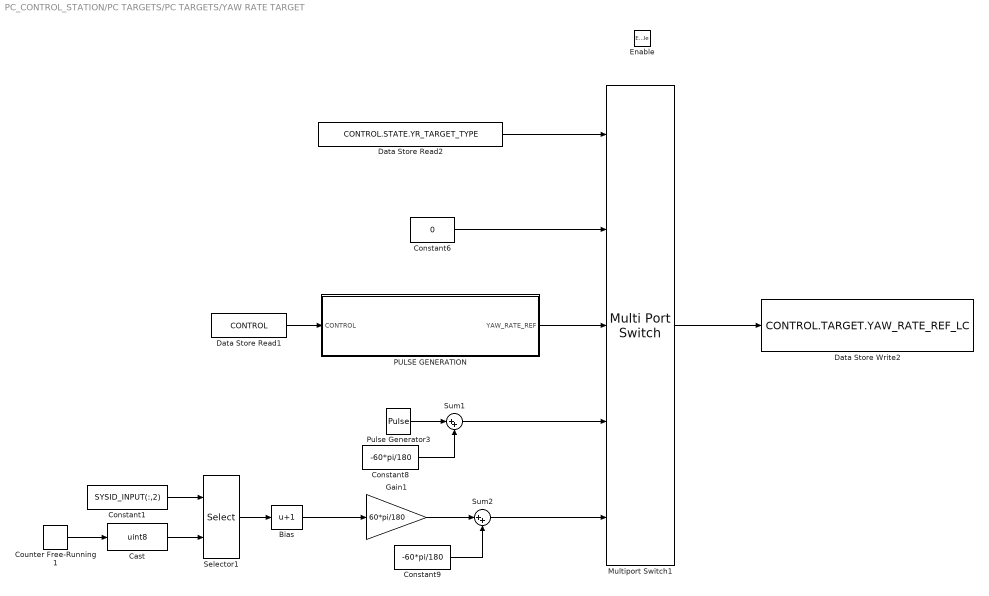
== system PC_CONTROL_STATION/PC TARGETS/PC TARGETS/YAW RATE TARGET ==
  Enable : EnablePort
  " PULSE GENERATION " : MATLAB Function  Priority=60  TreatAsAtomicUnit=on
  Bias : Bias  Bias=1  SaturateOnIntegerOverflow=off
  Cast : DataTypeConversion  OutDataTypeStr=uint8  SaturateOnIntegerOverflow=off  RndMeth=Floor
  Constant1 : Constant  Value=SYSID_INPUT(:,2)  SampleTime=SAMPLING_TIME
  Constant6 : Constant  Value=0  OutDataTypeStr=double  SampleTime=SAMPLING_TIME
  Constant8 : Constant  Value=-60*pi/180  OutDataTypeStr=single  SampleTime=SAMPLING_TIME
  Constant9 : Constant  Value=-60*pi/180  OutDataTypeStr=single  SampleTime=SAMPLING_TIME
  Counter Free-Running1 : simulink/Sources/Counter Free-Running  NumBits=9  tsamp=SAMPLING_TIME
  Data Store Read1 : DataStoreRead  DataStoreName=CONTROL  SampleTime=SAMPLING_TIME  IndexOptions=Index vector (dialog)  Indices=1  OutputSizes=1
  Data Store Read2 : DataStoreRead  DataStoreName=CONTROL  SampleTime=SAMPLING_TIME  DataStoreElements=CONTROL.STATE.YR_TARGET_TYPE  IndexOptions=Index vector (dialog)  Indices=1  OutputSizes=1
  Data Store Write2 : DataStoreWrite  DataStoreName=CONTROL  SampleTime=SAMPLING_TIME  DataStoreElements=CONTROL.TARGET.YAW_RATE_REF_LC  IndexOptions=Index vector (dialog)  Indices=1  OutputSizes=1
  Gain1 : Gain  Gain=60*pi/180
  Multiport Switch1 : MultiPortSwitch  DataPortOrder=Zero-based contiguous  Inputs=4  zeroidx=on  SaturateOnIntegerOverflow=off  InputSameDT=off
  Pulse Generator3 : DiscretePulseGenerator  Amplitude=120*pi/180  Period=500  PulseWidth=250  PhaseDelay=125  SampleTime=SAMPLING_TIME
  Selector1 : Selector  IndexMode=Zero-based  InputPortWidth=512  IndexOptions=Index vector (port)  Indices=[1 3]  OutputSizes=1
  Sum1 : Sum  Inputs=|++
  Sum2 : Sum  Inputs=|++
  wires:
  Sum2/1 -> Multiport Switch1/5
  Data Store Read2/1 -> Multiport Switch1/1
  Constant1/1 -> Selector1/1
  Multiport Switch1/1 -> Data Store Write2/1
  Constant6/1 -> Multiport Switch1/2
  Counter Free-Running1/1 -> Cast/1
  Cast/1 -> Selector1/2
  Data Store Read1/1 -> " PULSE GENERATION "/1(CONTROL)
  " PULSE GENERATION "/1(YAW_RATE_REF) -> Multiport Switch1/3
  Constant8/1 -> Sum1/2
  Constant9/1 -> Sum2/2
  Pulse Generator3/1 -> Sum1/1
  Selector1/1 -> Bias/1
  Sum1/1 -> Multiport Switch1/4
  Gain1/1 -> Sum2/1
  Bias/1 -> Gain1/1

== system PC_CONTROL_STATION/HARDWARE/RT_MONITORING/TCP 101/MSG_RX ==
  Bus Assignment : BusAssignment  AssignedSignals=RX_BUFFER
  Data Store Read : DataStoreRead  DataStoreName=MSG  IndexOptions=Index vector (dialog)  Indices=1  OutputSizes=1
  Data Store Write1 : DataStoreWrite  DataStoreName=MSG  IndexOptions=Index vector (dialog)  Indices=1  OutputSizes=1
  Packet Input : sldrtlib/Packet Input  SampleTime=CONTROL_INI.PARAM.COMM_SAMPLING_TIME  MaxMissedTicks=50  ShowMissedTicks=off  YieldWhenWaiting=off  DrvName=Standard_Devices/TCP_Protocol  DrvAddress=27001  DrvOptions=[0 27000 49 57 50 46 49 54 56 46 48 46 49 48 49 0 0 0 0 0 0 0 0 0 0 0 0 0 0 0 0 0 0 0 0 0 0 0 0 0 0 0 0 0 0 0 0 0 0 0 0 0 0 0 0 0 0 0 0 0 0 0 0 0 0 0 0 0 0 0 0 0 0 0 0 0 0 0 0 0 0 0 0 0 0 0 0 0 0 0 0 0 0 0 0 0 0 0 0 0 0 0 0 0 0 0 0 0 0 0 0 0 0 0 0 0 0 0 0 0 0 0 0 0 0 0 0 0 0 0 0 0 0 0 0 0 0 0 0 0 0 0 0 0 0 0 0 0 0 0 0 0 0 0 0 0 0 0 0 0 0 0 0 0 0 0 0 0 0 0 0 0 0 0 0 0 0 0 0 0 0 0 0 0 0 0 0 0 0 0 0 0 0 0 0 0 0 0 0 0 0 0 0 0 0 0 0 0 0 0 0 0 0 0 0 0 0 0 0 0 0 0 0 0 0 0 0 0 0 0 0 0 0 0 0 0 0 0 0 0 0 0 0 0 0 0 0 0 0 0 0 0 0 0 0 0]  PacketSize=1400  DataTypes={'1400*uint8'}  ShowReady=off  ShowError=off  PacketID=1  ByteOrder=2  ShowTimestamp=off
      settings: AttributesFormatString=TCP Protocol [27001]
  wires:
  Bus Assignment/1 -> Data Store Write1/1
  Data Store Read/1 -> Bus Assignment/1
  Packet Input/1 -> Bus Assignment/2

== system PC_CONTROL_STATION/HARDWARE/RT_MONITORING/TCP 101/MSG_TX  ==
  Enable : EnablePort
  Data Store Read1 : DataStoreRead  DataStoreName=MSG  DataStoreElements=MSG.TX_BUFFER(:,1)  IndexOptions=Index vector (dialog)  Indices=1  OutputSizes=1
  Packet Output : sldrtlib/Packet Output  SampleTime=CONTROL_INI.PARAM.COMM_SAMPLING_TIME  MaxMissedTicks=50  ShowMissedTicks=off  YieldWhenWaiting=off  DrvName=Standard_Devices/TCP_Protocol  DrvAddress=27000  DrvOptions=[0 27001 49 57 50 46 49 54 56 46 48 46 49 48 49 0 0 0 0 0 0 0 0 0 0 0 0 0 0 0 0 0 0 0 0 0 0 0 0 0 0 0 0 0 0 0 0 0 0 0 0 0 0 0 0 0 0 0 0 0 0 0 0 0 0 0 0 0 0 0 0 0 0 0 0 0 0 0 0 0 0 0 0 0 0 0 0 0 0 0 0 0 0 0 0 0 0 0 0 0 0 0 0 0 0 0 0 0 0 0 0 0 0 0 0 0 0 0 0 0 0 0 0 0 0 0 0 0 0 0 0 0 0 0 0 0 0 0 0 0 0 0 0 0 0 0 0 0 0 0 0 0 0 0 0 0 0 0 0 0 0 0 0 0 0 0 0 0 0 0 0 0 0 0 0 0 0 0 0 0 0 0 0 0 0 0 0 0 0 0 0 0 0 0 0 0 0 0 0 0 0 0 0 0 0 0 0 0 0 0 0 0 0 0 0 0 0 0 0 0 0 0 0 0 0 0 0 0 0 0 0 0 0 0 0 0 0 0 0 0 0 0 0 0 0 0 0 0 0 0 0 0 0 0 0 0]  PacketSize=1400  DataTypes={'1400*uint8'}  ShowReady=off  ShowError=off  PacketID=1  ByteOrder=2  InitialValue=[]  FinalValue=[]
      settings: AttributesFormatString=TCP Protocol [27000]
  wires:
  Data Store Read1/1 -> Packet Output/1

== system PC_CONTROL_STATION/HARDWARE/RT_MONITORING/TCP 102/MSG_RX ==
  Bus Assignment : BusAssignment  AssignedSignals=RX_BUFFER
  Data Store Read : DataStoreRead  DataStoreName=MSG  IndexOptions=Index vector (dialog)  Indices=1  OutputSizes=1
  Data Store Write1 : DataStoreWrite  DataStoreName=MSG  IndexOptions=Index vector (dialog)  Indices=1  OutputSizes=1
  Packet Input : sldrtlib/Packet Input  SampleTime=CONTROL_INI.PARAM.COMM_SAMPLING_TIME  MaxMissedTicks=50  ShowMissedTicks=off  YieldWhenWaiting=off  DrvName=Standard_Devices/TCP_Protocol  DrvAddress=27001  DrvOptions=[0 27000 49 57 50 46 49 54 56 46 48 46 49 48 50 0 0 0 0 0 0 0 0 0 0 0 0 0 0 0 0 0 0 0 0 0 0 0 0 0 0 0 0 0 0 0 0 0 0 0 0 0 0 0 0 0 0 0 0 0 0 0 0 0 0 0 0 0 0 0 0 0 0 0 0 0 0 0 0 0 0 0 0 0 0 0 0 0 0 0 0 0 0 0 0 0 0 0 0 0 0 0 0 0 0 0 0 0 0 0 0 0 0 0 0 0 0 0 0 0 0 0 0 0 0 0 0 0 0 0 0 0 0 0 0 0 0 0 0 0 0 0 0 0 0 0 0 0 0 0 0 0 0 0 0 0 0 0 0 0 0 0 0 0 0 0 0 0 0 0 0 0 0 0 0 0 0 0 0 0 0 0 0 0 0 0 0 0 0 0 0 0 0 0 0 0 0 0 0 0 0 0 0 0 0 0 0 0 0 0 0 0 0 0 0 0 0 0 0 0 0 0 0 0 0 0 0 0 0 0 0 0 0 0 0 0 0 0 0 0 0 0 0 0 0 0 0 0 0 0 0 0 0 0 0 0]  PacketSize=1400  DataTypes={'1400*uint8'}  ShowReady=off  ShowError=off  PacketID=1  ByteOrder=2  ShowTimestamp=off
      settings: AttributesFormatString=TCP Protocol [27001]
  wires:
  Bus Assignment/1 -> Data Store Write1/1
  Data Store Read/1 -> Bus Assignment/1
  Packet Input/1 -> Bus Assignment/2

== system PC_CONTROL_STATION/HARDWARE/RT_MONITORING/TCP 102/MSG_TX  ==
  Enable : EnablePort
  Data Store Read1 : DataStoreRead  DataStoreName=MSG  SampleTime=CONTROL_INI.PARAM.COMM_SAMPLING_TIME  DataStoreElements=MSG.TX_BUFFER(:,1)  IndexOptions=Index vector (dialog)  Indices=1  OutputSizes=1
  Packet Output : sldrtlib/Packet Output  SampleTime=CONTROL_INI.PARAM.COMM_SAMPLING_TIME  MaxMissedTicks=50  ShowMissedTicks=off  YieldWhenWaiting=off  DrvName=Standard_Devices/TCP_Protocol  DrvAddress=27000  DrvOptions=[0 27001 49 57 50 46 49 54 56 46 48 46 49 48 50 0 0 0 0 0 0 0 0 0 0 0 0 0 0 0 0 0 0 0 0 0 0 0 0 0 0 0 0 0 0 0 0 0 0 0 0 0 0 0 0 0 0 0 0 0 0 0 0 0 0 0 0 0 0 0 0 0 0 0 0 0 0 0 0 0 0 0 0 0 0 0 0 0 0 0 0 0 0 0 0 0 0 0 0 0 0 0 0 0 0 0 0 0 0 0 0 0 0 0 0 0 0 0 0 0 0 0 0 0 0 0 0 0 0 0 0 0 0 0 0 0 0 0 0 0 0 0 0 0 0 0 0 0 0 0 0 0 0 0 0 0 0 0 0 0 0 0 0 0 0 0 0 0 0 0 0 0 0 0 0 0 0 0 0 0 0 0 0 0 0 0 0 0 0 0 0 0 0 0 0 0 0 0 0 0 0 0 0 0 0 0 0 0 0 0 0 0 0 0 0 0 0 0 0 0 0 0 0 0 0 0 0 0 0 0 0 0 0 0 0 0 0 0 0 0 0 0 0 0 0 0 0 0 0 0 0 0 0 0 0 0]  PacketSize=1400  DataTypes={'1400*uint8'}  ShowReady=off  ShowError=off  PacketID=1  ByteOrder=2  InitialValue=[]  FinalValue=[]
      settings: AttributesFormatString=TCP Protocol [27000]
  wires:
  Data Store Read1/1 -> Packet Output/1

== system PC_CONTROL_STATION/HARDWARE/RT_MONITORING/TCP 103/MSG_RX ==
  Bus Assignment : BusAssignment  AssignedSignals=RX_BUFFER
  Data Store Read : DataStoreRead  DataStoreName=MSG  IndexOptions=Index vector (dialog)  Indices=1  OutputSizes=1
  Data Store Write1 : DataStoreWrite  DataStoreName=MSG  IndexOptions=Index vector (dialog)  Indices=1  OutputSizes=1
  Packet Input : sldrtlib/Packet Input  SampleTime=CONTROL_INI.PARAM.COMM_SAMPLING_TIME  MaxMissedTicks=50  ShowMissedTicks=off  YieldWhenWaiting=off  DrvName=Standard_Devices/TCP_Protocol  DrvAddress=27001  DrvOptions=[0 27000 49 57 50 46 49 54 56 46 48 46 49 48 51 0 0 0 0 0 0 0 0 0 0 0 0 0 0 0 0 0 0 0 0 0 0 0 0 0 0 0 0 0 0 0 0 0 0 0 0 0 0 0 0 0 0 0 0 0 0 0 0 0 0 0 0 0 0 0 0 0 0 0 0 0 0 0 0 0 0 0 0 0 0 0 0 0 0 0 0 0 0 0 0 0 0 0 0 0 0 0 0 0 0 0 0 0 0 0 0 0 0 0 0 0 0 0 0 0 0 0 0 0 0 0 0 0 0 0 0 0 0 0 0 0 0 0 0 0 0 0 0 0 0 0 0 0 0 0 0 0 0 0 0 0 0 0 0 0 0 0 0 0 0 0 0 0 0 0 0 0 0 0 0 0 0 0 0 0 0 0 0 0 0 0 0 0 0 0 0 0 0 0 0 0 0 0 0 0 0 0 0 0 0 0 0 0 0 0 0 0 0 0 0 0 0 0 0 0 0 0 0 0 0 0 0 0 0 0 0 0 0 0 0 0 0 0 0 0 0 0 0 0 0 0 0 0 0 0 0 0 0 0 0 0]  PacketSize=1400  DataTypes={'1400*uint8'}  ShowReady=off  ShowError=off  PacketID=1  ByteOrder=2  ShowTimestamp=off
      settings: AttributesFormatString=TCP Protocol [27001]
  wires:
  Bus Assignment/1 -> Data Store Write1/1
  Data Store Read/1 -> Bus Assignment/1
  Packet Input/1 -> Bus Assignment/2

== system PC_CONTROL_STATION/HARDWARE/RT_MONITORING/TCP 103/MSG_TX  ==
  Enable : EnablePort
  Data Store Read1 : DataStoreRead  DataStoreName=MSG  SampleTime=CONTROL_INI.PARAM.COMM_SAMPLING_TIME  DataStoreElements=MSG.TX_BUFFER(:,1)  IndexOptions=Index vector (dialog)  Indices=1  OutputSizes=1
  Packet Output : sldrtlib/Packet Output  SampleTime=CONTROL_INI.PARAM.COMM_SAMPLING_TIME  MaxMissedTicks=50  ShowMissedTicks=off  YieldWhenWaiting=off  DrvName=Standard_Devices/TCP_Protocol  DrvAddress=27000  DrvOptions=[0 27001 49 57 50 46 49 54 56 46 48 46 49 48 51 0 0 0 0 0 0 0 0 0 0 0 0 0 0 0 0 0 0 0 0 0 0 0 0 0 0 0 0 0 0 0 0 0 0 0 0 0 0 0 0 0 0 0 0 0 0 0 0 0 0 0 0 0 0 0 0 0 0 0 0 0 0 0 0 0 0 0 0 0 0 0 0 0 0 0 0 0 0 0 0 0 0 0 0 0 0 0 0 0 0 0 0 0 0 0 0 0 0 0 0 0 0 0 0 0 0 0 0 0 0 0 0 0 0 0 0 0 0 0 0 0 0 0 0 0 0 0 0 0 0 0 0 0 0 0 0 0 0 0 0 0 0 0 0 0 0 0 0 0 0 0 0 0 0 0 0 0 0 0 0 0 0 0 0 0 0 0 0 0 0 0 0 0 0 0 0 0 0 0 0 0 0 0 0 0 0 0 0 0 0 0 0 0 0 0 0 0 0 0 0 0 0 0 0 0 0 0 0 0 0 0 0 0 0 0 0 0 0 0 0 0 0 0 0 0 0 0 0 0 0 0 0 0 0 0 0 0 0 0 0 0]  PacketSize=1400  DataTypes={'1400*uint8'}  ShowReady=off  ShowError=off  PacketID=1  ByteOrder=2  InitialValue=[]  FinalValue=[]
      settings: AttributesFormatString=TCP Protocol [27000]
  wires:
  Data Store Read1/1 -> Packet Output/1

== system PC_CONTROL_STATION/HARDWARE/RT_MONITORING/TCP 104/MSG_RX ==
  Bus Assignment : BusAssignment  AssignedSignals=RX_BUFFER
  Data Store Read : DataStoreRead  DataStoreName=MSG  IndexOptions=Index vector (dialog)  Indices=1  OutputSizes=1
  Data Store Write1 : DataStoreWrite  DataStoreName=MSG  IndexOptions=Index vector (dialog)  Indices=1  OutputSizes=1
  Packet Input : sldrtlib/Packet Input  SampleTime=CONTROL_INI.PARAM.COMM_SAMPLING_TIME  MaxMissedTicks=50  ShowMissedTicks=off  YieldWhenWaiting=off  DrvName=Standard_Devices/TCP_Protocol  DrvAddress=27001  DrvOptions=[0 27000 49 57 50 46 49 54 56 46 48 46 49 48 52 0 0 0 0 0 0 0 0 0 0 0 0 0 0 0 0 0 0 0 0 0 0 0 0 0 0 0 0 0 0 0 0 0 0 0 0 0 0 0 0 0 0 0 0 0 0 0 0 0 0 0 0 0 0 0 0 0 0 0 0 0 0 0 0 0 0 0 0 0 0 0 0 0 0 0 0 0 0 0 0 0 0 0 0 0 0 0 0 0 0 0 0 0 0 0 0 0 0 0 0 0 0 0 0 0 0 0 0 0 0 0 0 0 0 0 0 0 0 0 0 0 0 0 0 0 0 0 0 0 0 0 0 0 0 0 0 0 0 0 0 0 0 0 0 0 0 0 0 0 0 0 0 0 0 0 0 0 0 0 0 0 0 0 0 0 0 0 0 0 0 0 0 0 0 0 0 0 0 0 0 0 0 0 0 0 0 0 0 0 0 0 0 0 0 0 0 0 0 0 0 0 0 0 0 0 0 0 0 0 0 0 0 0 0 0 0 0 0 0 0 0 0 0 0 0 0 0 0 0 0 0 0 0 0 0 0 0 0 0 0 0]  PacketSize=1400  DataTypes={'1400*uint8'}  ShowReady=off  ShowError=off  PacketID=1  ByteOrder=2  ShowTimestamp=off
      settings: AttributesFormatString=TCP Protocol [27001]
  wires:
  Bus Assignment/1 -> Data Store Write1/1
  Data Store Read/1 -> Bus Assignment/1
  Packet Input/1 -> Bus Assignment/2

== system PC_CONTROL_STATION/HARDWARE/RT_MONITORING/TCP 104/MSG_TX  ==
  Enable : EnablePort
  Data Store Read1 : DataStoreRead  DataStoreName=MSG  SampleTime=CONTROL_INI.PARAM.COMM_SAMPLING_TIME  DataStoreElements=MSG.TX_BUFFER(:,1)  IndexOptions=Index vector (dialog)  Indices=1  OutputSizes=1
  Packet Output : sldrtlib/Packet Output  SampleTime=CONTROL_INI.PARAM.COMM_SAMPLING_TIME  MaxMissedTicks=50  ShowMissedTicks=off  YieldWhenWaiting=off  DrvName=Standard_Devices/TCP_Protocol  DrvAddress=27000  DrvOptions=[0 27001 49 57 50 46 49 54 56 46 48 46 49 48 52 0 0 0 0 0 0 0 0 0 0 0 0 0 0 0 0 0 0 0 0 0 0 0 0 0 0 0 0 0 0 0 0 0 0 0 0 0 0 0 0 0 0 0 0 0 0 0 0 0 0 0 0 0 0 0 0 0 0 0 0 0 0 0 0 0 0 0 0 0 0 0 0 0 0 0 0 0 0 0 0 0 0 0 0 0 0 0 0 0 0 0 0 0 0 0 0 0 0 0 0 0 0 0 0 0 0 0 0 0 0 0 0 0 0 0 0 0 0 0 0 0 0 0 0 0 0 0 0 0 0 0 0 0 0 0 0 0 0 0 0 0 0 0 0 0 0 0 0 0 0 0 0 0 0 0 0 0 0 0 0 0 0 0 0 0 0 0 0 0 0 0 0 0 0 0 0 0 0 0 0 0 0 0 0 0 0 0 0 0 0 0 0 0 0 0 0 0 0 0 0 0 0 0 0 0 0 0 0 0 0 0 0 0 0 0 0 0 0 0 0 0 0 0 0 0 0 0 0 0 0 0 0 0 0 0 0 0 0 0 0 0]  PacketSize=1400  DataTypes={'1400*uint8'}  ShowReady=off  ShowError=off  PacketID=1  ByteOrder=2  InitialValue=[]  FinalValue=[]
      settings: AttributesFormatString=TCP Protocol [27000]
  wires:
  Data Store Read1/1 -> Packet Output/1

== system PC_CONTROL_STATION/HARDWARE/RT_MONITORING/TCP 105/MSG_RX ==
  Bus Assignment : BusAssignment  AssignedSignals=RX_BUFFER
  Data Store Read : DataStoreRead  DataStoreName=MSG  IndexOptions=Index vector (dialog)  Indices=1  OutputSizes=1
  Data Store Write1 : DataStoreWrite  DataStoreName=MSG  IndexOptions=Index vector (dialog)  Indices=1  OutputSizes=1
  Packet Input : sldrtlib/Packet Input  SampleTime=CONTROL_INI.PARAM.COMM_SAMPLING_TIME  MaxMissedTicks=50  ShowMissedTicks=off  YieldWhenWaiting=off  DrvName=Standard_Devices/TCP_Protocol  DrvAddress=27001  DrvOptions=[0 27000 49 57 50 46 49 54 56 46 48 46 49 48 53 0 0 0 0 0 0 0 0 0 0 0 0 0 0 0 0 0 0 0 0 0 0 0 0 0 0 0 0 0 0 0 0 0 0 0 0 0 0 0 0 0 0 0 0 0 0 0 0 0 0 0 0 0 0 0 0 0 0 0 0 0 0 0 0 0 0 0 0 0 0 0 0 0 0 0 0 0 0 0 0 0 0 0 0 0 0 0 0 0 0 0 0 0 0 0 0 0 0 0 0 0 0 0 0 0 0 0 0 0 0 0 0 0 0 0 0 0 0 0 0 0 0 0 0 0 0 0 0 0 0 0 0 0 0 0 0 0 0 0 0 0 0 0 0 0 0 0 0 0 0 0 0 0 0 0 0 0 0 0 0 0 0 0 0 0 0 0 0 0 0 0 0 0 0 0 0 0 0 0 0 0 0 0 0 0 0 0 0 0 0 0 0 0 0 0 0 0 0 0 0 0 0 0 0 0 0 0 0 0 0 0 0 0 0 0 0 0 0 0 0 0 0 0 0 0 0 0 0 0 0 0 0 0 0 0 0 0 0 0 0 0]  PacketSize=1400  DataTypes={'1400*uint8'}  ShowReady=off  ShowError=off  PacketID=1  ByteOrder=2  ShowTimestamp=off
      settings: AttributesFormatString=TCP Protocol [27001]
  wires:
  Bus Assignment/1 -> Data Store Write1/1
  Data Store Read/1 -> Bus Assignment/1
  Packet Input/1 -> Bus Assignment/2

== system PC_CONTROL_STATION/HARDWARE/RT_MONITORING/TCP 105/MSG_TX  ==
  Enable : EnablePort
  Data Store Read1 : DataStoreRead  DataStoreName=MSG  SampleTime=CONTROL_INI.PARAM.COMM_SAMPLING_TIME  DataStoreElements=MSG.TX_BUFFER(:,1)  IndexOptions=Index vector (dialog)  Indices=1  OutputSizes=1
  Packet Output : sldrtlib/Packet Output  SampleTime=CONTROL_INI.PARAM.COMM_SAMPLING_TIME  MaxMissedTicks=50  ShowMissedTicks=off  YieldWhenWaiting=off  DrvName=Standard_Devices/TCP_Protocol  DrvAddress=27000  DrvOptions=[0 27001 49 57 50 46 49 54 56 46 48 46 49 48 53 0 0 0 0 0 0 0 0 0 0 0 0 0 0 0 0 0 0 0 0 0 0 0 0 0 0 0 0 0 0 0 0 0 0 0 0 0 0 0 0 0 0 0 0 0 0 0 0 0 0 0 0 0 0 0 0 0 0 0 0 0 0 0 0 0 0 0 0 0 0 0 0 0 0 0 0 0 0 0 0 0 0 0 0 0 0 0 0 0 0 0 0 0 0 0 0 0 0 0 0 0 0 0 0 0 0 0 0 0 0 0 0 0 0 0 0 0 0 0 0 0 0 0 0 0 0 0 0 0 0 0 0 0 0 0 0 0 0 0 0 0 0 0 0 0 0 0 0 0 0 0 0 0 0 0 0 0 0 0 0 0 0 0 0 0 0 0 0 0 0 0 0 0 0 0 0 0 0 0 0 0 0 0 0 0 0 0 0 0 0 0 0 0 0 0 0 0 0 0 0 0 0 0 0 0 0 0 0 0 0 0 0 0 0 0 0 0 0 0 0 0 0 0 0 0 0 0 0 0 0 0 0 0 0 0 0 0 0 0 0 0]  PacketSize=1400  DataTypes={'1400*uint8'}  ShowReady=off  ShowError=off  PacketID=1  ByteOrder=2  InitialValue=[]  FinalValue=[]
      settings: AttributesFormatString=TCP Protocol [27000]
  wires:
  Data Store Read1/1 -> Packet Output/1

== system PC_CONTROL_STATION/HARDWARE/RT_MONITORING/TCP 106/MSG_RX ==
  Bus Assignment : BusAssignment  AssignedSignals=RX_BUFFER
  Data Store Read : DataStoreRead  DataStoreName=MSG  IndexOptions=Index vector (dialog)  Indices=1  OutputSizes=1
  Data Store Write1 : DataStoreWrite  DataStoreName=MSG  IndexOptions=Index vector (dialog)  Indices=1  OutputSizes=1
  Packet Input : sldrtlib/Packet Input  SampleTime=CONTROL_INI.PARAM.COMM_SAMPLING_TIME  MaxMissedTicks=50  ShowMissedTicks=off  YieldWhenWaiting=off  DrvName=Standard_Devices/TCP_Protocol  DrvAddress=27001  DrvOptions=[0 27000 49 57 50 46 49 54 56 46 48 46 49 48 54 0 0 0 0 0 0 0 0 0 0 0 0 0 0 0 0 0 0 0 0 0 0 0 0 0 0 0 0 0 0 0 0 0 0 0 0 0 0 0 0 0 0 0 0 0 0 0 0 0 0 0 0 0 0 0 0 0 0 0 0 0 0 0 0 0 0 0 0 0 0 0 0 0 0 0 0 0 0 0 0 0 0 0 0 0 0 0 0 0 0 0 0 0 0 0 0 0 0 0 0 0 0 0 0 0 0 0 0 0 0 0 0 0 0 0 0 0 0 0 0 0 0 0 0 0 0 0 0 0 0 0 0 0 0 0 0 0 0 0 0 0 0 0 0 0 0 0 0 0 0 0 0 0 0 0 0 0 0 0 0 0 0 0 0 0 0 0 0 0 0 0 0 0 0 0 0 0 0 0 0 0 0 0 0 0 0 0 0 0 0 0 0 0 0 0 0 0 0 0 0 0 0 0 0 0 0 0 0 0 0 0 0 0 0 0 0 0 0 0 0 0 0 0 0 0 0 0 0 0 0 0 0 0 0 0 0 0 0 0 0 0]  PacketSize=1400  DataTypes={'1400*uint8'}  ShowReady=off  ShowError=off  PacketID=1  ByteOrder=2  ShowTimestamp=off
      settings: AttributesFormatString=TCP Protocol [27001]
  wires:
  Bus Assignment/1 -> Data Store Write1/1
  Data Store Read/1 -> Bus Assignment/1
  Packet Input/1 -> Bus Assignment/2
